simulink model "PMSG2"  (Simulink 8.1)
settings: Solver=ode45  StartTime=0.0  StopTime=50  RelTol=1e-3
libraries: simulink x2
settings Model: Creator=korichi  LastModifiedBy=apple
settings OptimizationCC: InitFltsAndDblsToZero=on
settings DebuggingCC: StrictBusMsg=Warning

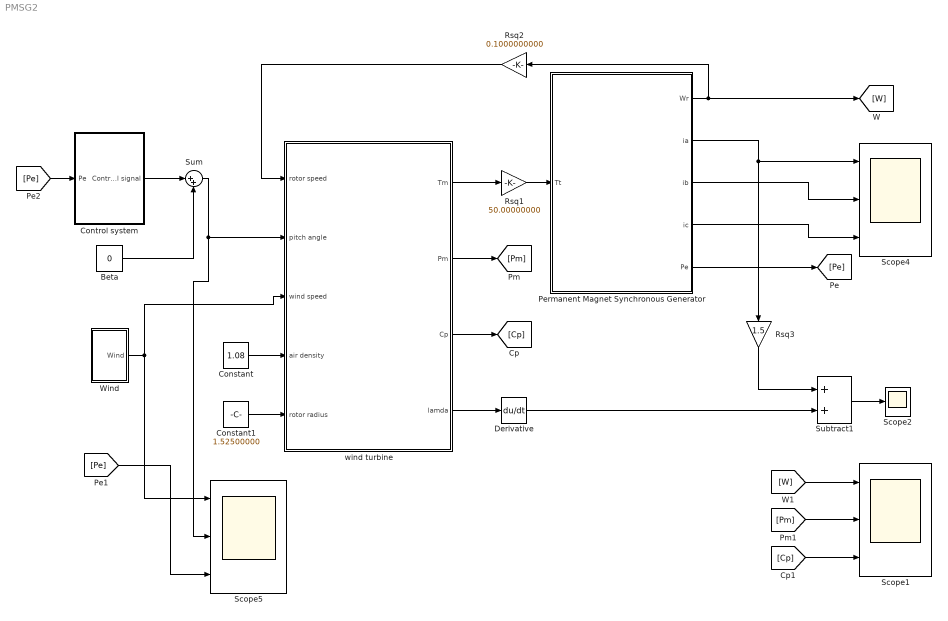
== system PMSG2 ==
  Beta : Constant  Value=0
  Constant : Constant  Value=1.08
  Constant1 : Constant  Value=1.52500000
  Control system : Subsystem
  Derivative : Derivative
  Permanent Magnet Synchronous Generator : Subsystem
  Rsq1 : Gain  Gain=50.00000000
  Rsq2 : Gain  Gain=0.1000000000
  Rsq3 : Gain  Gain=1.5
  Scope1 : Scope  NumInputPorts=3
      settings: YMin=44.7~25.25~0.0187  YMax=46.3~27.75~0.0205  SaveName=TeW2  MaxDataPoints=100000000
  Scope2 : Scope
      settings: TimeRange=10  YMin=-9  YMax=9  SaveName=TeW  MaxDataPoints=100000000  SampleInput=on
  Scope4 : Scope  NumInputPorts=3
      settings: YMin=-0.7~-0.7~-0.7  YMax=0.7~0.7~0.7  SaveName=TeW6  MaxDataPoints=100000000
  Scope5 : Scope  NumInputPorts=3
      settings: TimeRange=10  YMin=17~-5~-5  YMax=17.07~5~5  SaveName=TeW7  MaxDataPoints=100000000  SampleInput=on
  Subtract1 : Sum
  Sum : Sum  Inputs=|++
  Wind : Subsystem
  wind turbine : Subsystem
  wires:
  Constant/1 -> wind turbine/4(air density)
  Constant1/1 -> wind turbine/5(rotor radius)
  wind turbine/1(Tm) -> Rsq1/1
  Rsq2/1 -> wind turbine/1(rotor speed)
  Rsq1/1 -> Permanent Magnet Synchronous Generator/1(Tt)
  wind turbine/3(Cp) -> [Cp]
  wind turbine/2(Pm) -> [Pm]
  [Cp] -> Scope1/3
  [Pm] -> Scope1/2
  [W] -> Scope1/1
  Permanent Magnet Synchronous Generator/2(ia) -> Scope4/1, Rsq3/1
  Rsq3/1 -> Subtract1/1
  wind turbine/4(lamda) -> Derivative/1
  Derivative/1 -> Subtract1/2
  Permanent Magnet Synchronous Generator/1(Wr) -> [W], Rsq2/1
  Subtract1/1 -> Scope2/1
  Permanent Magnet Synchronous Generator/3(ib) -> Scope4/2
  Permanent Magnet Synchronous Generator/4(ic) -> Scope4/3
  Wind/1(Wind) -> Scope5/1, wind turbine/3(wind speed)
  Permanent Magnet Synchronous Generator/5(Pe) -> [Pe]
  Beta/1 -> Sum/2
  Sum/1 -> wind turbine/2(pitch angle), Scope5/2
  [Pe] -> Scope5/3
  [Pe] -> Control system/1(Pe)
  Control system/1(Control signal) -> Sum/1

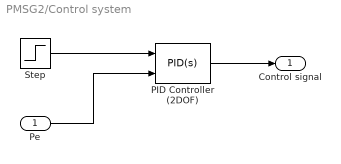
== system PMSG2/Control system ==
  Pe : Inport
  PID Controller (2DOF) : simulink/Continuous/PID Controller (2DOF)  Controller=PID  TimeDomain=Continuous-time  SampleTime=1  IntegratorMethod=Forward Euler  FilterMethod=Forward Euler  Form=Parallel  P=18.5288128227141  I=86.5967997347677  D=0.610070474760475  N=21.9186219727111  b=1  c=1  InitialConditionSource=internal  InitialConditionForIntegrator=0  InitialConditionForFilter=0  ExternalReset=none  LimitOutput=on  UpperSaturationLimit=90  LowerSaturationLimit=0  LinearizeAsGain=on  AntiWindupMode=clamping  Kb=1  TrackingMode=off  Kt=1  PParamMin=[]  PParamMax=[]  IParamMin=[]  IParamMax=[]  DParamMin=[]  DParamMax=[]  NParamMin=[]  NParamMax=[]  bParamMin=[]  bParamMax=[]  cParamMin=[]  cParamMax=[]  KbParamMin=[]  KbParamMax=[]  KtParamMin=[]  KtParamMax=[]  POutMin=[]  POutMax=[]  IOutMin=[]  IOutMax=[]  DOutMin=[]  DOutMax=[]  NOutMin=[]  NOutMax=[]  bOutMin=[]  bOutMax=[]  cOutMin=[]  cOutMax=[]  KbOutMin=[]  KbOutMax=[]  KtOutMin=[]  KtOutMax=[]  IntegratorOutMin=[]  IntegratorOutMax=[]  FilterOutMin=[]  FilterOutMax=[]  SumOutMin=[]  SumOutMax=[]  Sum1OutMin=[]  Sum1OutMax=[]  Sum2OutMin=[]  Sum2OutMax=[]  Sum3OutMin=[]  Sum3OutMax=[]  SumI1OutMin=[]  SumI1OutMax=[]  SumI2OutMin=[]  SumI2OutMax=[]  SumI3OutMin=[]  SumI3OutMax=[]  SumDOutMin=[]  SumDOutMax=[]  SaturationOutMin=[]  SaturationOutMax=[]  IntegratorContinuousStateAttributes=''  IntegratorStateMustResolveToSignalObject=off  IntegratorRTWStateStorageClass=Auto  FilterContinuousStateAttributes=''  FilterStateMustResolveToSignalObject=off  FilterRTWStateStorageClass=Auto
  Step : Step  After=14  SampleTime=0
  Control signal : Outport
  wires:
  PID Controller (2DOF)/1 -> Control signal/1
  Step/1 -> PID Controller (2DOF)/1
  Pe/1 -> PID Controller (2DOF)/2

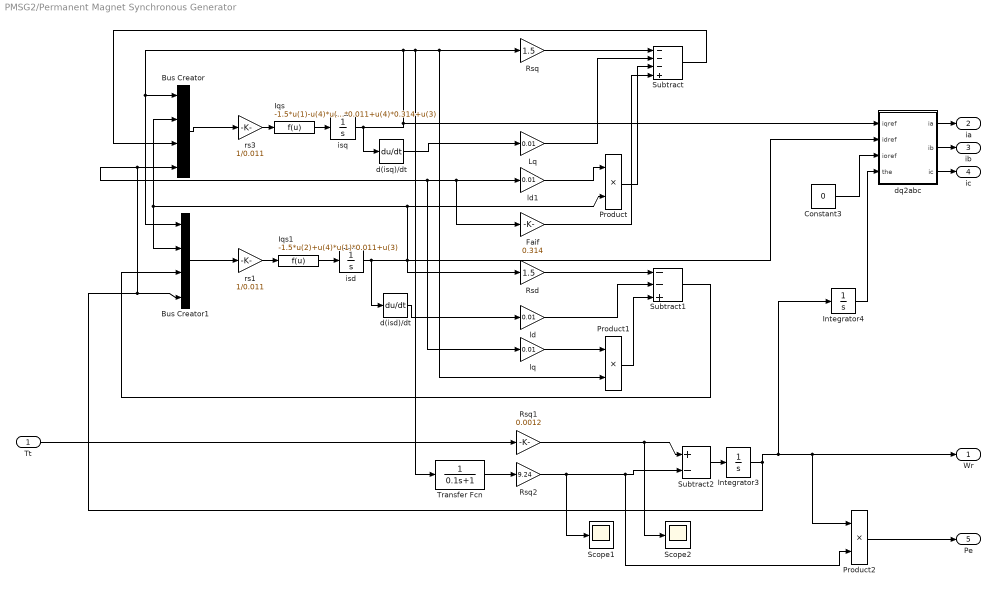
== system PMSG2/Permanent Magnet Synchronous Generator ==
  Tt : Inport
  Bus Creator : BusCreator
  Bus Creator1 : BusCreator
  Constant3 : Constant  Value=0
  Faif : Gain  Gain=0.314
  Integrator3 : Integrator  InitialCondition=1  IgnoreLimit=on
  Integrator4 : Integrator
  Iqs : Fcn  Expr=-1.5*u(1)-u(4)*u(2)*0.011+u(4)*0.314+u(3)
  Iqs1 : Fcn  Expr=-1.5*u(2)+u(4)*u(1)*0.011+u(3)
  Lq : Gain  Gain=0.01
  Product : Product  RndMeth=Zero
  Product1 : Product  RndMeth=Zero
  Product2 : Product  RndMeth=Zero
  Rsd : Gain  Gain=1.5
  Rsq : Gain  Gain=1.5
  Rsq1 : Gain  Gain=0.0012
  Rsq2 : Gain  Gain=9.24
  Scope1 : Scope
      settings: TimeRange=10  YMin=0.65  YMax=1.4  SaveName=TeW5  MaxDataPoints=100000000  SampleInput=on
  Scope2 : Scope
      settings: TimeRange=10  YMin=-30  YMax=15  SaveName=TeW4  MaxDataPoints=100000000  SampleInput=on
  Subtract : Sum  Inputs=---+
  Subtract1 : Sum  Inputs=--+
  Subtract2 : Sum  Inputs=+-
  Transfer Fcn : TransferFcn  Denominator=[0.1 1]
  d(isd)/dt : Derivative
  d(isq)/dt : Derivative
  dq2abc : Subsystem
  isd : Integrator
  isq : Integrator
  ld : Gain  Gain=0.01
  ld1 : Gain  Gain=0.01
  lq : Gain  Gain=0.01
  rs1 : Gain  Gain=1/0.011
  rs3 : Gain  Gain=1/0.011
  Wr : Outport
  ia : Outport  Port=2
  ib : Outport  Port=3
  ic : Outport  Port=4
  Pe : Outport  Port=5
  wires:
  Rsq/1 -> Subtract/1
  Iqs/1 -> isq/1
  rs3/1 -> Iqs/1
  Bus Creator/1 -> rs3/1
  Rsq1/1 -> Scope2/1, Subtract2/1
  Rsq2/1 -> Scope1/1, Product2/2, Subtract2/2
  Subtract2/1 -> Integrator3/1
  Iqs1/1 -> isd/1
  rs1/1 -> Iqs1/1
  Bus Creator1/1 -> rs1/1
  Constant3/1 -> dq2abc/3(ioref)
  dq2abc/1(ia) -> ia/1
  isq/1 -> Bus Creator/1, Bus Creator1/1, Transfer Fcn/1, Product1/2, Rsq/1, dq2abc/1(iqref), d(isq)/dt/1
  isd/1 -> Bus Creator/2, Bus Creator1/2, Product/2, dq2abc/2(idref), Rsd/1, d(isd)/dt/1
  Lq/1 -> Subtract/2
  ld1/1 -> Product/1
  Product/1 -> Subtract/3
  Faif/1 -> Subtract/4
  Rsd/1 -> Subtract1/1
  ld/1 -> Subtract1/2
  Subtract/1 -> Bus Creator/3
  lq/1 -> Product1/1
  Product1/1 -> Subtract1/3
  Subtract1/1 -> Bus Creator1/3
  Tt/1 -> Rsq1/1
  Integrator3/1 -> Wr/1, Product2/1, Integrator4/1, Bus Creator1/4, Bus Creator/4, ld1/1, Faif/1, lq/1
  d(isq)/dt/1 -> Lq/1
  d(isd)/dt/1 -> ld/1
  Integrator4/1 -> dq2abc/4(the)
  dq2abc/2(ib) -> ib/1
  dq2abc/3(ic) -> ic/1
  Product2/1 -> Pe/1
  Transfer Fcn/1 -> Rsq2/1

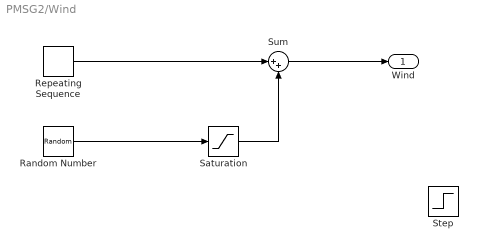
== system PMSG2/Wind ==
  Random Number : RandomNumber  Seed=20  SampleTime=0
  Repeating Sequence : simulink/Sources/Repeating Sequence  rep_seq_t=[0 2]  rep_seq_y=[0 2]
  Saturation : Saturate  UpperLimit=12  LowerLimit=5
  Step : Step  After=2  SampleTime=0
  Sum : Sum  Inputs=|++
  Wind : Outport
  wires:
  Random Number/1 -> Saturation/1
  Saturation/1 -> Sum/2
  Sum/1 -> Wind/1
  Repeating Sequence/1 -> Sum/1

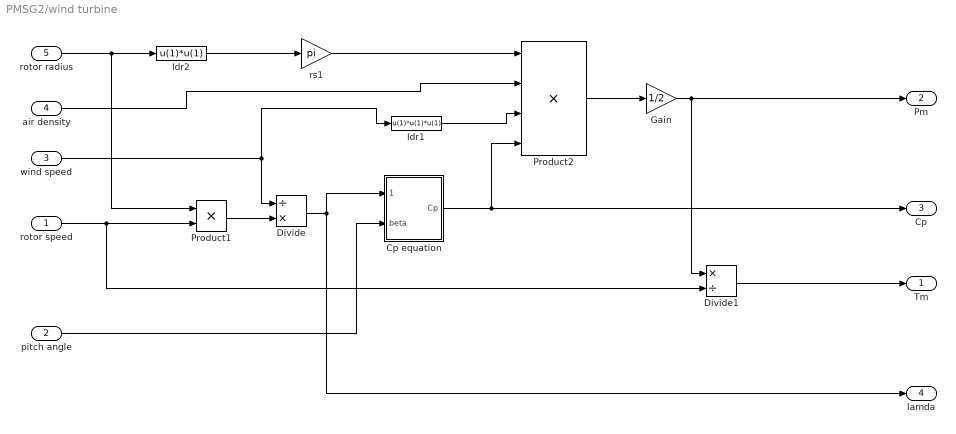
== system PMSG2/wind turbine ==
  rotor speed : Inport
  pitch angle : Inport  Port=2
  wind speed : Inport  Port=3
  air density : Inport  Port=4
  rotor radius : Inport  Port=5
  Cp equation : Subsystem
  Divide : Product  Inputs=/*
  Divide1 : Product  Inputs=*/
  Gain : Gain  Gain=1/2
  Idr1 : Fcn  Expr=u(1)*u(1)*u(1)
  Idr2 : Fcn  Expr=u(1)*u(1)
  Product1 : Product  RndMeth=Zero
  Product2 : Product  Inputs=4  RndMeth=Zero
  rs1 : Gain  Gain=pi
  Tm : Outport
  Pm : Outport  Port=2
  Cp : Outport  Port=3
  lamda : Outport  Port=4
  wires:
  Cp equation/1(Cp) -> Product2/4, Cp/1
  Divide/1 -> Cp equation/1(lambda), lamda/1
  rotor speed/1 -> Product1/2, Divide1/2
  Gain/1 -> Divide1/1, Pm/1
  air density/1 -> Product2/2
  Idr1/1 -> Product2/3
  Product2/1 -> Gain/1
  rotor radius/1 -> Product1/1, Idr2/1
  wind speed/1 -> Idr1/1, Divide/1
  Product1/1 -> Divide/2
  rs1/1 -> Product2/1
  Idr2/1 -> rs1/1
  Divide1/1 -> Tm/1
  pitch angle/1 -> Cp equation/2(beta)

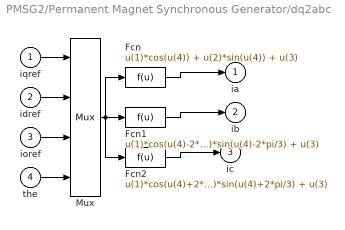
== system PMSG2/Permanent Magnet Synchronous Generator/dq2abc ==
  iqref : Inport
  idref : Inport  Port=2
  ioref : Inport  Port=3
  the : Inport  Port=4
  Fcn : Fcn  Expr=u(1)*cos(u(4)) + u(2)*sin(u(4)) + u(3)
  Fcn1 : Fcn  Expr=u(1)*cos(u(4)-2*pi/3) + u(2)*sin(u(4)-2*pi/3) + u(3)
  Fcn2 : Fcn  Expr=u(1)*cos(u(4)+2*pi/3)+ u(2)*sin(u(4)+2*pi/3) + u(3)
  Mux : Mux
  ia : Outport  InitialOutput=0
  ib : Outport  Port=2  InitialOutput=0
  ic : Outport  Port=3  InitialOutput=0
  wires:
  the/1 -> Mux/4
  ioref/1 -> Mux/3
  idref/1 -> Mux/2
  iqref/1 -> Mux/1
  Mux/1 -> Fcn1/1, Fcn2/1, Fcn/1
  Fcn1/1 -> ib/1
  Fcn/1 -> ia/1
  Fcn2/1 -> ic/1

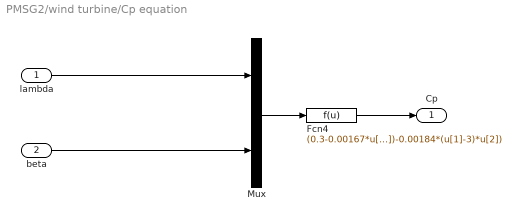
== system PMSG2/wind turbine/Cp equation ==
  lambda : Inport
  beta : Inport  Port=2
  Fcn4 : Fcn  Expr=(0.3-0.00167*u[2])*sin(pi*(u[1]+0.1)/(10-0.3*u[2])-0.00184*(u[1]-3)*u[2])
  Mux : Mux  Inputs=2
  Cp : Outport
  wires:
  beta/1 -> Mux/2
  lambda/1 -> Mux/1
  Fcn4/1 -> Cp/1
  Mux/1 -> Fcn4/1
